simulink model "pet_logical_architecture"  (R2024a)
settings: Solver=FixedStepDiscrete  StartTime=0.0  StopTime=10.0  RelTol=1e-3
settings Model: Creator=diell  LastModifiedBy=diell

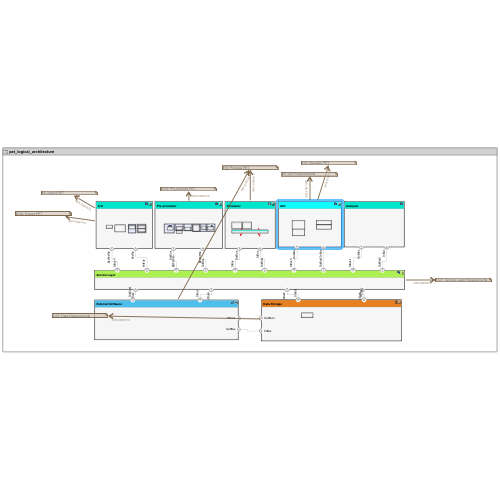
[thumbnail: Simulink's stored preview of the top-level diagram]
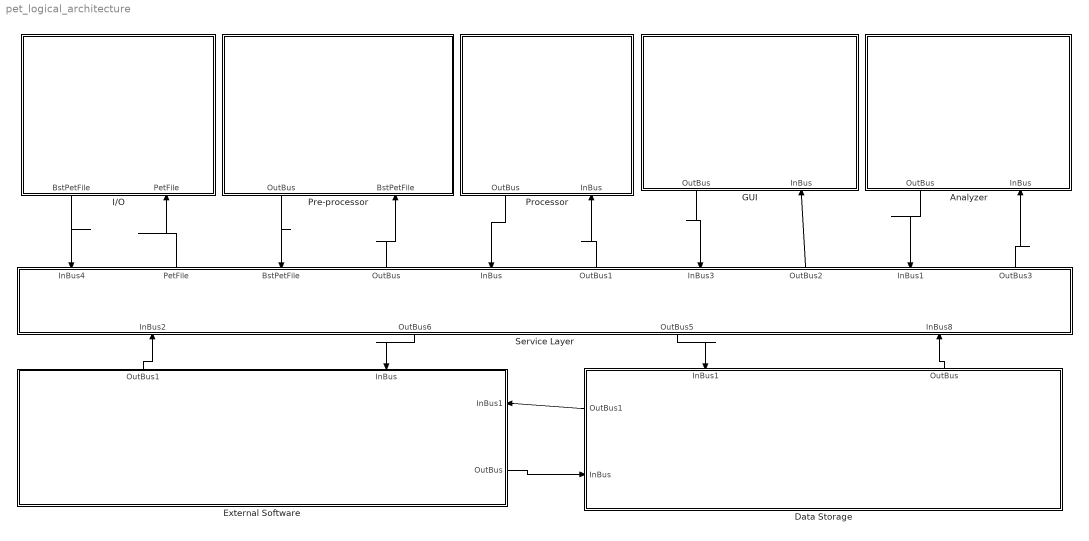
== system pet_logical_architecture ==
  Analyzer : Subsystem
      settings: PortSchema="{\"entries\":[{\"content\":{\"headerSize\":26,\"margin\":15,\"minimumSpacing\":25,\"sides\":[{\"content\":{},\"type\":\"ConnectorPlacement.EquallySpacedRectSide\",\"uuid\":\"231a4a51-e9d6-4ee1-a9d5-4e29b655c305\"},{\"content\":{\"side\":\"RIGHT\"},\"type\":\"ConnectorPlacement.EquallySpacedRectSide\",\"uuid\":\"e9ceff5f-0784-495f-ae83-524709d043d6\"},{\"content\":{\"side\":\"TOP\"},\"type\":\"ConnectorPlacement.EquallySpacedRectSide\",\"uuid\":\"01c193fb-23d5-46fa-9f50-f56eecaefc77\"},{\"content\":{\"connectorIds\":[\"Out1\",\"In1\"],\"side\":\"BOTTOM\"},\"type\":\"ConnectorPlacement.EquallySpacedRectSide\",\"uuid\":\"6027dc84-36e6-4171-8066-96bc152a4b70\"}]},\"type\":\"ConnectorPlacement.EquallySpacedConnector\",\"uuid\":\"bc597724-759a-481a-a480-4165a84a707f\"}],\"packageUris\":[\"http://schema.mathworks.com/mf0/Connector/R2020b\"],\"version\":\"1.0\"}"
  Data Storage : Subsystem
      settings: PortSchema="{\"entries\":[{\"content\":{\"headerSize\":26,\"margin\":15,\"minimumSpacing\":25,\"sides\":[{\"content\":{\"connectorIds\":[\"Out1\",\"In1\"]},\"type\":\"ConnectorPlacement.EquallySpacedRectSide\",\"uuid\":\"231a4a51-e9d6-4ee1-a9d5-4e29b655c305\"},{\"content\":{\"side\":\"RIGHT\"},\"type\":\"ConnectorPlacement.EquallySpacedRectSide\",\"uuid\":\"e9ceff5f-0784-495f-ae83-524709d043d6\"},{\"content\":{\"connectorIds\":[\"In2\",\"Out2\"],\"side\":\"TOP\"},\"type\":\"ConnectorPlacement.EquallySpacedRectSide\",\"uuid\":\"01c193fb-23d5-46fa-9f50-f56eecaefc77\"}]},\"type\":\"ConnectorPlacement.EquallySpacedConnector\",\"uuid\":\"bc597724-759a-481a-a480-4165a84a707f\"}],\"packageUris\":[\"http://schema.mathworks.com/mf0/Connector/R2020b\"],\"version\":\"1.0\"}"
  External Software : Subsystem
      settings: PortSchema="{\"entries\":[{\"content\":{\"headerSize\":26,\"margin\":15,\"minimumSpacing\":25,\"sides\":[{\"content\":{},\"type\":\"ConnectorPlacement.EquallySpacedRectSide\",\"uuid\":\"231a4a51-e9d6-4ee1-a9d5-4e29b655c305\"},{\"content\":{\"connectorIds\":[\"In1\",\"Out1\"],\"side\":\"RIGHT\"},\"type\":\"ConnectorPlacement.EquallySpacedRectSide\",\"uuid\":\"e9ceff5f-0784-495f-ae83-524709d043d6\"},{\"content\":{\"connectorIds\":[\"Out2\",\"In2\"],\"side\":\"TOP\"},\"type\":\"ConnectorPlacement.EquallySpacedRectSide\",\"uuid\":\"01c193fb-23d5-46fa-9f50-f56eecaefc77\"}]},\"type\":\"ConnectorPlacement.EquallySpacedConnector\",\"uuid\":\"bc597724-759a-481a-a480-4165a84a707f\"}],\"packageUris\":[\"http://schema.mathworks.com/mf0/Connector/R2020b\"],\"version\":\"1.0\"}"
  GUI : Subsystem
      settings: PortSchema="{\"entries\":[{\"content\":{\"headerSize\":26,\"margin\":15,\"minimumSpacing\":25,\"sides\":[{\"content\":{},\"type\":\"ConnectorPlacement.EquallySpacedRectSide\",\"uuid\":\"231a4a51-e9d6-4ee1-a9d5-4e29b655c305\"},{\"content\":{\"side\":\"RIGHT\"},\"type\":\"ConnectorPlacement.EquallySpacedRectSide\",\"uuid\":\"e9ceff5f-0784-495f-ae83-524709d043d6\"},{\"content\":{\"side\":\"TOP\"},\"type\":\"ConnectorPlacement.EquallySpacedRectSide\",\"uuid\":\"01c193fb-23d5-46fa-9f50-f56eecaefc77\"},{\"content\":{\"connectorIds\":[\"Out1\",\"In1\"],\"side\":\"BOTTOM\"},\"type\":\"ConnectorPlacement.EquallySpacedRectSide\",\"uuid\":\"8789287b-37dd-46ec-841a-db569d1bc1a9\"}]},\"type\":\"ConnectorPlacement.EquallySpacedConnector\",\"uuid\":\"bc597724-759a-481a-a480-4165a84a707f\"}],\"packageUris\":[\"http://schema.mathworks.com/mf0/Connector/R2020b\"],\"version\":\"1.0\"}"
  "I/O " : Subsystem
      settings: PortSchema="{\"entries\":[{\"content\":{\"headerSize\":26,\"margin\":15,\"minimumSpacing\":25,\"sides\":[{\"content\":{},\"type\":\"ConnectorPlacement.EquallySpacedRectSide\",\"uuid\":\"231a4a51-e9d6-4ee1-a9d5-4e29b655c305\"},{\"content\":{\"side\":\"RIGHT\"},\"type\":\"ConnectorPlacement.EquallySpacedRectSide\",\"uuid\":\"e9ceff5f-0784-495f-ae83-524709d043d6\"},{\"content\":{\"side\":\"TOP\"},\"type\":\"ConnectorPlacement.EquallySpacedRectSide\",\"uuid\":\"01c193fb-23d5-46fa-9f50-f56eecaefc77\"},{\"content\":{\"connectorIds\":[\"Out1\",\"In1\"],\"side\":\"BOTTOM\"},\"type\":\"ConnectorPlacement.EquallySpacedRectSide\",\"uuid\":\"53c8788b-6d16-4a86-bf5b-c8def0072bdd\"}]},\"type\":\"ConnectorPlacement.EquallySpacedConnector\",\"uuid\":\"bc597724-759a-481a-a480-4165a84a707f\"}],\"packageUris\":[\"http://schema.mathworks.com/mf0/Connector/R2020b\"],\"version\":\"1.0\"}"
  Pre-processor : Subsystem
      settings: PortSchema="{\"entries\":[{\"content\":{\"headerSize\":26,\"margin\":15,\"minimumSpacing\":25,\"sides\":[{\"content\":{},\"type\":\"ConnectorPlacement.EquallySpacedRectSide\",\"uuid\":\"231a4a51-e9d6-4ee1-a9d5-4e29b655c305\"},{\"content\":{\"side\":\"RIGHT\"},\"type\":\"ConnectorPlacement.EquallySpacedRectSide\",\"uuid\":\"e9ceff5f-0784-495f-ae83-524709d043d6\"},{\"content\":{\"side\":\"TOP\"},\"type\":\"ConnectorPlacement.EquallySpacedRectSide\",\"uuid\":\"01c193fb-23d5-46fa-9f50-f56eecaefc77\"},{\"content\":{\"connectorIds\":[\"Out1\",\"In1\"],\"side\":\"BOTTOM\"},\"type\":\"ConnectorPlacement.EquallySpacedRectSide\",\"uuid\":\"b0b0d034-7ae8-4ce9-aa3d-1431a9441512\"}]},\"type\":\"ConnectorPlacement.EquallySpacedConnector\",\"uuid\":\"bc597724-759a-481a-a480-4165a84a707f\"}],\"packageUris\":[\"http://schema.mathworks.com/mf0/Connector/R2020b\"],\"version\":\"1.0\"}"
  Processor : Subsystem
      settings: PortSchema="{\"entries\":[{\"content\":{\"headerSize\":26,\"margin\":15,\"minimumSpacing\":25,\"sides\":[{\"content\":{},\"type\":\"ConnectorPlacement.EquallySpacedRectSide\",\"uuid\":\"231a4a51-e9d6-4ee1-a9d5-4e29b655c305\"},{\"content\":{\"side\":\"RIGHT\"},\"type\":\"ConnectorPlacement.EquallySpacedRectSide\",\"uuid\":\"e9ceff5f-0784-495f-ae83-524709d043d6\"},{\"content\":{\"side\":\"TOP\"},\"type\":\"ConnectorPlacement.EquallySpacedRectSide\",\"uuid\":\"01c193fb-23d5-46fa-9f50-f56eecaefc77\"},{\"content\":{\"connectorIds\":[\"Out1\",\"In1\"],\"side\":\"BOTTOM\"},\"type\":\"ConnectorPlacement.EquallySpacedRectSide\",\"uuid\":\"096d348b-1de6-4ed0-877f-8a116cb4ec66\"}]},\"type\":\"ConnectorPlacement.EquallySpacedConnector\",\"uuid\":\"bc597724-759a-481a-a480-4165a84a707f\"}],\"packageUris\":[\"http://schema.mathworks.com/mf0/Connector/R2020b\"],\"version\":\"1.0\"}"
  Service Layer : Subsystem
      settings: PortSchema="{\"entries\":[{\"content\":{\"headerSize\":26,\"margin\":15,\"minimumSpacing\":25,\"sides\":[{\"content\":{},\"type\":\"ConnectorPlacement.EquallySpacedRectSide\",\"uuid\":\"231a4a51-e9d6-4ee1-a9d5-4e29b655c305\"},{\"content\":{\"side\":\"RIGHT\"},\"type\":\"ConnectorPlacement.EquallySpacedRectSide\",\"uuid\":\"e9ceff5f-0784-495f-ae83-524709d043d6\"},{\"content\":{\"connectorIds\":[\"In1\",\"Out1\",\"In5\",\"Out3\",\"In2\",\"Out2\",\"In3\",\"Out4\",\"In4\",\"Out5\"],\"side\":\"TOP\"},\"type\":\"ConnectorPlacement.EquallySpacedRectSide\",\"uuid\":\"01c193fb-23d5-46fa-9f50-f56eecaefc77\"},{\"content\":{\"connectorIds\":[\"In6\",\"Out6\",\"Out7\",\"In7\"],\"side\":\"BOTTOM\"},\"type\":\"ConnectorPlacement.EquallySpacedRectSide\",\"uuid\":\"8a7a1846-1a54-4dcd-b18c-069e384b1e61\"}]},\"type\":\"ConnectorPlacement.EquallySpacedConnector\",\"uuid\":\"bc597724-759a-481a-a480-4165a84a707f\"}],\"packageUris\":[\"http://schema.mathworks.com/mf0/Connector/R2020b\"],\"version\":\"1.0\"}"
  wires:
  Data Storage/2(OutBus) -> Service Layer/7(InBus8)
  Service Layer/7(OutBus5) -> Data Storage/2(InBus1)
  Service Layer/6(OutBus6) -> External Software/2(InBus)
  External Software/2(OutBus1) -> Service Layer/6(InBus2)
  External Software/1(OutBus) -> Data Storage/1(InBus)
  Data Storage/1(OutBus1) -> External Software/1(InBus1)
  Service Layer/1(PetFile) -> "I/O "/1(PetFile)
  Pre-processor/1(OutBus) -> Service Layer/5(BstPetFile)
  Service Layer/3(OutBus) -> Pre-processor/1(BstPetFile)
  Processor/1(OutBus) -> Service Layer/2(InBus)
  Service Layer/2(OutBus1) -> Processor/1(InBus)
  GUI/1(OutBus) -> Service Layer/3(InBus3)
  Service Layer/4(OutBus2) -> GUI/1(InBus)
  Analyzer/1(OutBus) -> Service Layer/4(InBus1)
  Service Layer/5(OutBus3) -> Analyzer/1(InBus)
  "I/O "/1(BstPetFile) -> Service Layer/1(InBus4)

== system pet_logical_architecture/Analyzer ==
  Bus Element In1 : Inport  PortName=InBus
  Bus Element Out1 : Outport  PortName=OutBus

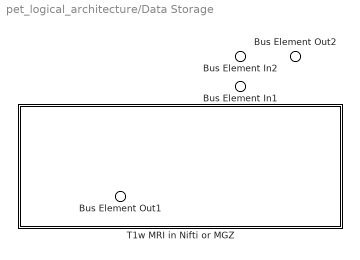
== system pet_logical_architecture/Data Storage ==
  Bus Element In1 : Inport  PortName=InBus
  Bus Element In2 : Inport  Port=2  PortName=InBus1
  T1w MRI in Nifti or MGZ : Subsystem
      settings: PortSchema="{\"entries\":[{\"content\":{\"headerSize\":26,\"margin\":15,\"minimumSpacing\":25,\"sides\":[{\"content\":{},\"type\":\"ConnectorPlacement.EquallySpacedRectSide\",\"uuid\":\"41d3ebd7-d990-4c64-a8fe-a1444a13acba\"},{\"content\":{\"side\":\"RIGHT\"},\"type\":\"ConnectorPlacement.EquallySpacedRectSide\",\"uuid\":\"34a032e5-8bdc-4c16-a398-56e9e8002181\"},{\"content\":{\"side\":\"TOP\"},\"type\":\"ConnectorPlacement.EquallySpacedRectSide\",\"uuid\":\"d28171cf-e891-45d3-8ea9-b10c38c32c2e\"}]},\"type\":\"ConnectorPlacement.EquallySpacedConnector\",\"uuid\":\"0daa939b-8979-496f-bab9-c42cbb494216\"}],\"packageUris\":[\"http://schema.mathworks.com/mf0/Connector/R2020b\"],\"version\":\"1.0\"}"
  Bus Element Out2 : Outport  PortName=OutBus1
  Bus Element Out1 : Outport  Port=2  PortName=OutBus

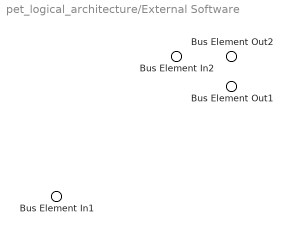
== system pet_logical_architecture/External Software ==
  Bus Element In2 : Inport  PortName=InBus1
  Bus Element In1 : Inport  Port=2  PortName=InBus
  Bus Element Out1 : Outport  PortName=OutBus
  Bus Element Out2 : Outport  Port=2  PortName=OutBus1

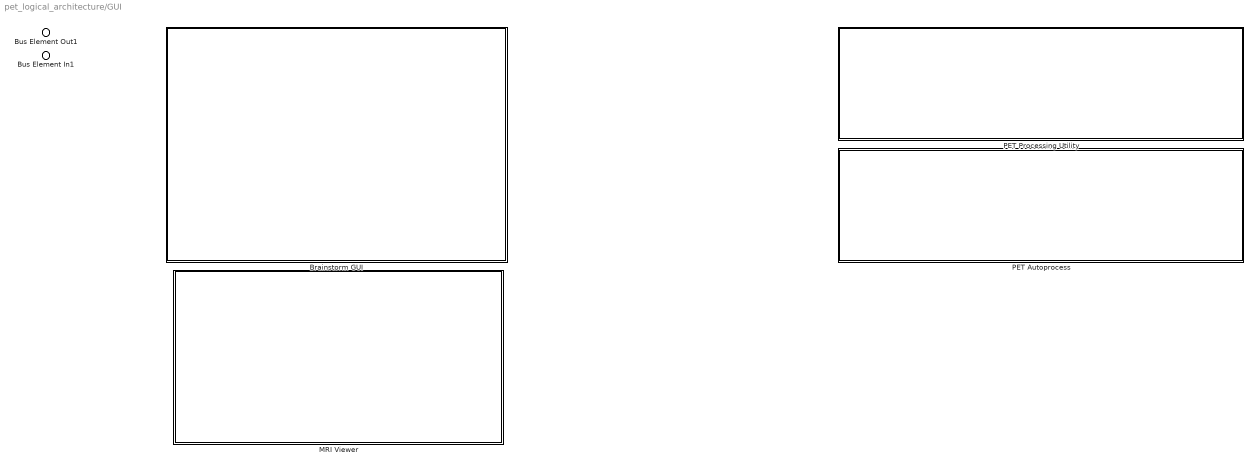
== system pet_logical_architecture/GUI ==
  Bus Element In1 : Inport  PortName=InBus
  "Brainstorm GUI " : Subsystem
      settings: PortSchema="{\"entries\":[{\"content\":{\"headerSize\":26,\"margin\":15,\"minimumSpacing\":25,\"sides\":[{\"content\":{},\"type\":\"ConnectorPlacement.EquallySpacedRectSide\",\"uuid\":\"41d3ebd7-d990-4c64-a8fe-a1444a13acba\"},{\"content\":{\"side\":\"RIGHT\"},\"type\":\"ConnectorPlacement.EquallySpacedRectSide\",\"uuid\":\"34a032e5-8bdc-4c16-a398-56e9e8002181\"},{\"content\":{\"side\":\"TOP\"},\"type\":\"ConnectorPlacement.EquallySpacedRectSide\",\"uuid\":\"d28171cf-e891-45d3-8ea9-b10c38c32c2e\"}]},\"type\":\"ConnectorPlacement.EquallySpacedConnector\",\"uuid\":\"0daa939b-8979-496f-bab9-c42cbb494216\"}],\"packageUris\":[\"http://schema.mathworks.com/mf0/Connector/R2020b\"],\"version\":\"1.0\"}"
  MRI Viewer : Subsystem
      settings: PortSchema="{\"entries\":[{\"content\":{\"headerSize\":26,\"margin\":15,\"minimumSpacing\":25,\"sides\":[{\"content\":{},\"type\":\"ConnectorPlacement.EquallySpacedRectSide\",\"uuid\":\"41d3ebd7-d990-4c64-a8fe-a1444a13acba\"},{\"content\":{\"side\":\"RIGHT\"},\"type\":\"ConnectorPlacement.EquallySpacedRectSide\",\"uuid\":\"34a032e5-8bdc-4c16-a398-56e9e8002181\"},{\"content\":{\"side\":\"TOP\"},\"type\":\"ConnectorPlacement.EquallySpacedRectSide\",\"uuid\":\"d28171cf-e891-45d3-8ea9-b10c38c32c2e\"}]},\"type\":\"ConnectorPlacement.EquallySpacedConnector\",\"uuid\":\"0daa939b-8979-496f-bab9-c42cbb494216\"}],\"packageUris\":[\"http://schema.mathworks.com/mf0/Connector/R2020b\"],\"version\":\"1.0\"}"
  PET Autoprocess : Subsystem
      settings: PortSchema="{\"entries\":[{\"content\":{\"headerSize\":26,\"margin\":15,\"minimumSpacing\":25,\"sides\":[{\"content\":{},\"type\":\"ConnectorPlacement.EquallySpacedRectSide\",\"uuid\":\"41d3ebd7-d990-4c64-a8fe-a1444a13acba\"},{\"content\":{\"side\":\"RIGHT\"},\"type\":\"ConnectorPlacement.EquallySpacedRectSide\",\"uuid\":\"34a032e5-8bdc-4c16-a398-56e9e8002181\"},{\"content\":{\"side\":\"TOP\"},\"type\":\"ConnectorPlacement.EquallySpacedRectSide\",\"uuid\":\"d28171cf-e891-45d3-8ea9-b10c38c32c2e\"}]},\"type\":\"ConnectorPlacement.EquallySpacedConnector\",\"uuid\":\"0daa939b-8979-496f-bab9-c42cbb494216\"}],\"packageUris\":[\"http://schema.mathworks.com/mf0/Connector/R2020b\"],\"version\":\"1.0\"}"
  PET Processing Utility : Subsystem
      settings: PortSchema="{\"entries\":[{\"content\":{\"headerSize\":26,\"margin\":15,\"minimumSpacing\":25,\"sides\":[{\"content\":{},\"type\":\"ConnectorPlacement.EquallySpacedRectSide\",\"uuid\":\"41d3ebd7-d990-4c64-a8fe-a1444a13acba\"},{\"content\":{\"side\":\"RIGHT\"},\"type\":\"ConnectorPlacement.EquallySpacedRectSide\",\"uuid\":\"34a032e5-8bdc-4c16-a398-56e9e8002181\"},{\"content\":{\"side\":\"TOP\"},\"type\":\"ConnectorPlacement.EquallySpacedRectSide\",\"uuid\":\"d28171cf-e891-45d3-8ea9-b10c38c32c2e\"}]},\"type\":\"ConnectorPlacement.EquallySpacedConnector\",\"uuid\":\"0daa939b-8979-496f-bab9-c42cbb494216\"}],\"packageUris\":[\"http://schema.mathworks.com/mf0/Connector/R2020b\"],\"version\":\"1.0\"}"
  Bus Element Out1 : Outport  PortName=OutBus

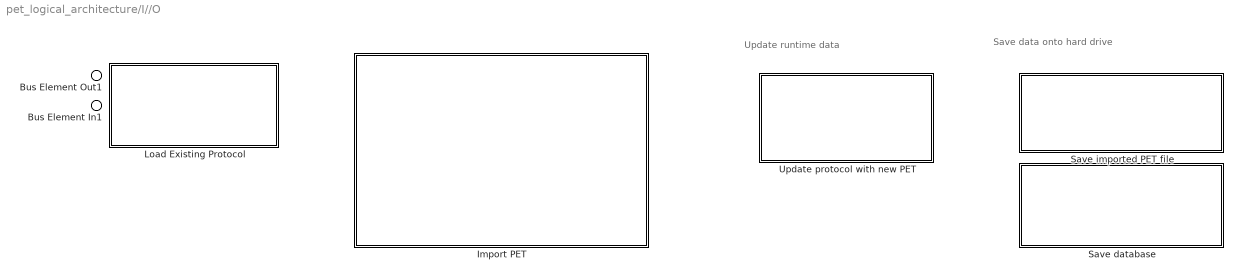
== system pet_logical_architecture/I//O  ==
  note: Save data onto hard drive
  note: Update runtime data
  Bus Element In1 : Inport  PortName=PetFile
  Import PET : Subsystem
      settings: PortSchema="{\"entries\":[{\"content\":{\"headerSize\":26,\"margin\":15,\"minimumSpacing\":25,\"sides\":[{\"content\":{},\"type\":\"ConnectorPlacement.EquallySpacedRectSide\",\"uuid\":\"9a42c3ee-f5d5-46c5-b9f0-29e49ed7c7b7\"},{\"content\":{\"side\":\"RIGHT\"},\"type\":\"ConnectorPlacement.EquallySpacedRectSide\",\"uuid\":\"669ba6ca-2a72-430e-84d2-b9b4202c74ab\"},{\"content\":{\"side\":\"TOP\"},\"type\":\"ConnectorPlacement.EquallySpacedRectSide\",\"uuid\":\"659c07dc-ee6b-4566-a70e-b6beb842b74e\"}]},\"type\":\"ConnectorPlacement.EquallySpacedConnector\",\"uuid\":\"e9499bf4-698a-44d7-8b3a-a6a8c827afce\"}],\"packageUris\":[\"http://schema.mathworks.com/mf0/Connector/R2020b\"],\"version\":\"1.0\"}"
  Load Existing Protocol : Subsystem
      settings: PortSchema="{\"entries\":[{\"content\":{\"headerSize\":26,\"margin\":15,\"minimumSpacing\":25,\"sides\":[{\"content\":{},\"type\":\"ConnectorPlacement.EquallySpacedRectSide\",\"uuid\":\"9a42c3ee-f5d5-46c5-b9f0-29e49ed7c7b7\"},{\"content\":{\"side\":\"RIGHT\"},\"type\":\"ConnectorPlacement.EquallySpacedRectSide\",\"uuid\":\"669ba6ca-2a72-430e-84d2-b9b4202c74ab\"},{\"content\":{\"side\":\"TOP\"},\"type\":\"ConnectorPlacement.EquallySpacedRectSide\",\"uuid\":\"659c07dc-ee6b-4566-a70e-b6beb842b74e\"}]},\"type\":\"ConnectorPlacement.EquallySpacedConnector\",\"uuid\":\"e9499bf4-698a-44d7-8b3a-a6a8c827afce\"}],\"packageUris\":[\"http://schema.mathworks.com/mf0/Connector/R2020b\"],\"version\":\"1.0\"}"
  Save database : Subsystem
      settings: PortSchema="{\"entries\":[{\"content\":{\"headerSize\":26,\"margin\":15,\"minimumSpacing\":25,\"sides\":[{\"content\":{},\"type\":\"ConnectorPlacement.EquallySpacedRectSide\",\"uuid\":\"9a42c3ee-f5d5-46c5-b9f0-29e49ed7c7b7\"},{\"content\":{\"side\":\"RIGHT\"},\"type\":\"ConnectorPlacement.EquallySpacedRectSide\",\"uuid\":\"669ba6ca-2a72-430e-84d2-b9b4202c74ab\"},{\"content\":{\"side\":\"TOP\"},\"type\":\"ConnectorPlacement.EquallySpacedRectSide\",\"uuid\":\"659c07dc-ee6b-4566-a70e-b6beb842b74e\"}]},\"type\":\"ConnectorPlacement.EquallySpacedConnector\",\"uuid\":\"e9499bf4-698a-44d7-8b3a-a6a8c827afce\"}],\"packageUris\":[\"http://schema.mathworks.com/mf0/Connector/R2020b\"],\"version\":\"1.0\"}"
  Save imported PET file : Subsystem
      settings: PortSchema="{\"entries\":[{\"content\":{\"headerSize\":26,\"margin\":15,\"minimumSpacing\":25,\"sides\":[{\"content\":{},\"type\":\"ConnectorPlacement.EquallySpacedRectSide\",\"uuid\":\"9a42c3ee-f5d5-46c5-b9f0-29e49ed7c7b7\"},{\"content\":{\"side\":\"RIGHT\"},\"type\":\"ConnectorPlacement.EquallySpacedRectSide\",\"uuid\":\"669ba6ca-2a72-430e-84d2-b9b4202c74ab\"},{\"content\":{\"side\":\"TOP\"},\"type\":\"ConnectorPlacement.EquallySpacedRectSide\",\"uuid\":\"659c07dc-ee6b-4566-a70e-b6beb842b74e\"}]},\"type\":\"ConnectorPlacement.EquallySpacedConnector\",\"uuid\":\"e9499bf4-698a-44d7-8b3a-a6a8c827afce\"}],\"packageUris\":[\"http://schema.mathworks.com/mf0/Connector/R2020b\"],\"version\":\"1.0\"}"
  Update protocol with new PET : Subsystem
      settings: PortSchema="{\"entries\":[{\"content\":{\"headerSize\":26,\"margin\":15,\"minimumSpacing\":25,\"sides\":[{\"content\":{},\"type\":\"ConnectorPlacement.EquallySpacedRectSide\",\"uuid\":\"9a42c3ee-f5d5-46c5-b9f0-29e49ed7c7b7\"},{\"content\":{\"side\":\"RIGHT\"},\"type\":\"ConnectorPlacement.EquallySpacedRectSide\",\"uuid\":\"669ba6ca-2a72-430e-84d2-b9b4202c74ab\"},{\"content\":{\"side\":\"TOP\"},\"type\":\"ConnectorPlacement.EquallySpacedRectSide\",\"uuid\":\"659c07dc-ee6b-4566-a70e-b6beb842b74e\"},{\"content\":{\"side\":\"BOTTOM\"},\"type\":\"ConnectorPlacement.EquallySpacedRectSide\",\"uuid\":\"cf282e21-1e43-4117-abb4-23de90c90cc3\"}]},\"type\":\"ConnectorPlacement.EquallySpacedConnector\",\"uuid\":\"e9499bf4-698a-44d7-8b3a-a6a8c827afce\"}],\"packageUris\":[\"http://schema.mathworks.com/mf0/Connector/R2020b\"],\"version\":\"1.0\"}"
  Bus Element Out1 : Outport  PortName=BstPetFile

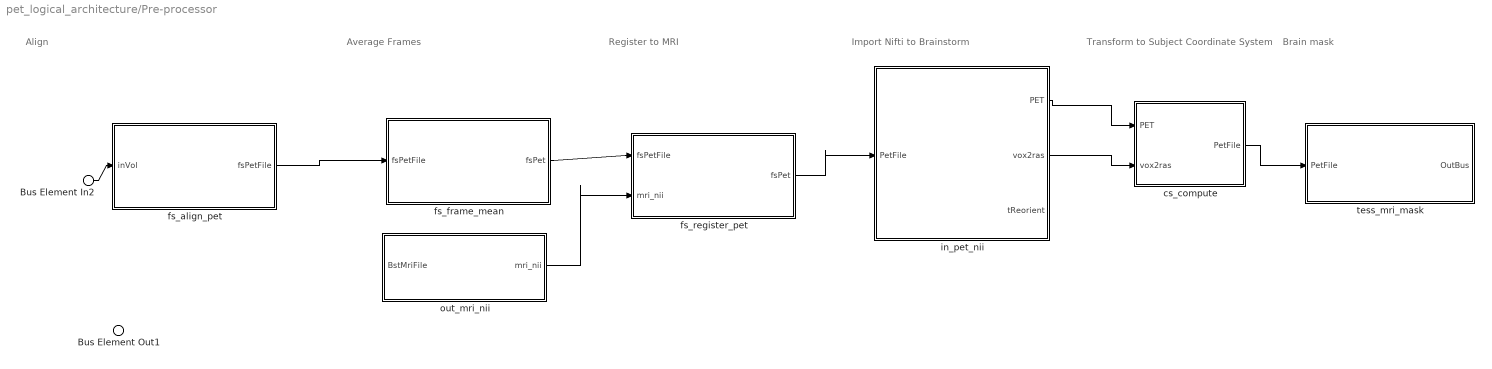
== system pet_logical_architecture/Pre-processor ==
  note: Align
  note: Average Frames
  note: Transform to
      | Subject Coordinate System
  note: Register to MRI
  note: Brain mask
  note: Import Nifti to Brainstorm
  Bus Element In2 : Inport  PortName=BstPetFile
  cs_compute : Subsystem
      settings: PortSchema="{\"entries\":[{\"content\":{\"headerSize\":26,\"margin\":15,\"minimumSpacing\":25,\"sides\":[{\"content\":{\"connectorIds\":[\"In1\",\"In2\"]},\"type\":\"ConnectorPlacement.EquallySpacedRectSide\",\"uuid\":\"d9face5b-155e-4e83-95c0-d581b737b6e3\"},{\"content\":{\"connectorIds\":[\"Out1\"],\"side\":\"RIGHT\"},\"type\":\"ConnectorPlacement.EquallySpacedRectSide\",\"uuid\":\"f965be1f-1639-4140-b9ea-f5e9efbe4150\"},{\"content\":{\"side\":\"TOP\"},\"type\":\"ConnectorPlacement.EquallySpacedRectSide\",\"uuid\":\"7c9c4b2b-011c-4482-afab-b6e67025a5e2\"}]},\"type\":\"ConnectorPlacement.EquallySpacedConnector\",\"uuid\":\"ec963004-117d-4f22-bb00-71f35201e6e2\"}],\"packageUris\":[\"http://schema.mathworks.com/mf0/Connector/R2020b\"],\"version\":\"1.0\"}"
  fs_align_pet : Subsystem
      settings: PortSchema="{\"entries\":[{\"content\":{\"headerSize\":26,\"margin\":15,\"minimumSpacing\":25,\"sides\":[{\"content\":{\"connectorIds\":[\"In1\"]},\"type\":\"ConnectorPlacement.EquallySpacedRectSide\",\"uuid\":\"d9face5b-155e-4e83-95c0-d581b737b6e3\"},{\"content\":{\"connectorIds\":[\"Out1\"],\"side\":\"RIGHT\"},\"type\":\"ConnectorPlacement.EquallySpacedRectSide\",\"uuid\":\"f965be1f-1639-4140-b9ea-f5e9efbe4150\"},{\"content\":{\"side\":\"TOP\"},\"type\":\"ConnectorPlacement.EquallySpacedRectSide\",\"uuid\":\"7c9c4b2b-011c-4482-afab-b6e67025a5e2\"}]},\"type\":\"ConnectorPlacement.EquallySpacedConnector\",\"uuid\":\"ec963004-117d-4f22-bb00-71f35201e6e2\"}],\"packageUris\":[\"http://schema.mathworks.com/mf0/Connector/R2020b\"],\"version\":\"1.0\"}"
  fs_frame_mean : Subsystem
      settings: PortSchema="{\"entries\":[{\"content\":{\"headerSize\":26,\"margin\":15,\"minimumSpacing\":25,\"sides\":[{\"content\":{\"connectorIds\":[\"In1\"]},\"type\":\"ConnectorPlacement.EquallySpacedRectSide\",\"uuid\":\"d9face5b-155e-4e83-95c0-d581b737b6e3\"},{\"content\":{\"connectorIds\":[\"Out1\"],\"side\":\"RIGHT\"},\"type\":\"ConnectorPlacement.EquallySpacedRectSide\",\"uuid\":\"f965be1f-1639-4140-b9ea-f5e9efbe4150\"},{\"content\":{\"side\":\"TOP\"},\"type\":\"ConnectorPlacement.EquallySpacedRectSide\",\"uuid\":\"7c9c4b2b-011c-4482-afab-b6e67025a5e2\"}]},\"type\":\"ConnectorPlacement.EquallySpacedConnector\",\"uuid\":\"ec963004-117d-4f22-bb00-71f35201e6e2\"}],\"packageUris\":[\"http://schema.mathworks.com/mf0/Connector/R2020b\"],\"version\":\"1.0\"}"
  fs_register_pet : Subsystem
      settings: PortSchema="{\"entries\":[{\"content\":{\"headerSize\":26,\"margin\":15,\"minimumSpacing\":25,\"sides\":[{\"content\":{\"connectorIds\":[\"In1\",\"In2\"]},\"type\":\"ConnectorPlacement.EquallySpacedRectSide\",\"uuid\":\"d9face5b-155e-4e83-95c0-d581b737b6e3\"},{\"content\":{\"connectorIds\":[\"Out1\"],\"side\":\"RIGHT\"},\"type\":\"ConnectorPlacement.EquallySpacedRectSide\",\"uuid\":\"f965be1f-1639-4140-b9ea-f5e9efbe4150\"},{\"content\":{\"side\":\"TOP\"},\"type\":\"ConnectorPlacement.EquallySpacedRectSide\",\"uuid\":\"7c9c4b2b-011c-4482-afab-b6e67025a5e2\"}]},\"type\":\"ConnectorPlacement.EquallySpacedConnector\",\"uuid\":\"ec963004-117d-4f22-bb00-71f35201e6e2\"}],\"packageUris\":[\"http://schema.mathworks.com/mf0/Connector/R2020b\"],\"version\":\"1.0\"}"
  in_pet_nii : Subsystem
      settings: PortSchema="{\"entries\":[{\"content\":{\"headerSize\":26,\"margin\":15,\"minimumSpacing\":25,\"sides\":[{\"content\":{\"connectorIds\":[\"In1\"]},\"type\":\"ConnectorPlacement.EquallySpacedRectSide\",\"uuid\":\"d9face5b-155e-4e83-95c0-d581b737b6e3\"},{\"content\":{\"connectorIds\":[\"Out1\",\"Out2\",\"Out3\"],\"side\":\"RIGHT\"},\"type\":\"ConnectorPlacement.EquallySpacedRectSide\",\"uuid\":\"f965be1f-1639-4140-b9ea-f5e9efbe4150\"},{\"content\":{\"side\":\"TOP\"},\"type\":\"ConnectorPlacement.EquallySpacedRectSide\",\"uuid\":\"7c9c4b2b-011c-4482-afab-b6e67025a5e2\"}]},\"type\":\"ConnectorPlacement.EquallySpacedConnector\",\"uuid\":\"ec963004-117d-4f22-bb00-71f35201e6e2\"}],\"packageUris\":[\"http://schema.mathworks.com/mf0/Connector/R2020b\"],\"version\":\"1.0\"}"
  out_mri_nii : Subsystem
      settings: PortSchema="{\"entries\":[{\"content\":{\"headerSize\":26,\"margin\":15,\"minimumSpacing\":25,\"sides\":[{\"content\":{\"connectorIds\":[\"In1\"]},\"type\":\"ConnectorPlacement.EquallySpacedRectSide\",\"uuid\":\"d9face5b-155e-4e83-95c0-d581b737b6e3\"},{\"content\":{\"connectorIds\":[\"Out1\"],\"side\":\"RIGHT\"},\"type\":\"ConnectorPlacement.EquallySpacedRectSide\",\"uuid\":\"f965be1f-1639-4140-b9ea-f5e9efbe4150\"},{\"content\":{\"side\":\"TOP\"},\"type\":\"ConnectorPlacement.EquallySpacedRectSide\",\"uuid\":\"7c9c4b2b-011c-4482-afab-b6e67025a5e2\"}]},\"type\":\"ConnectorPlacement.EquallySpacedConnector\",\"uuid\":\"ec963004-117d-4f22-bb00-71f35201e6e2\"}],\"packageUris\":[\"http://schema.mathworks.com/mf0/Connector/R2020b\"],\"version\":\"1.0\"}"
  tess_mri_mask : Subsystem
      settings: PortSchema="{\"entries\":[{\"content\":{\"headerSize\":26,\"margin\":15,\"minimumSpacing\":25,\"sides\":[{\"content\":{\"connectorIds\":[\"In1\"]},\"type\":\"ConnectorPlacement.EquallySpacedRectSide\",\"uuid\":\"d9face5b-155e-4e83-95c0-d581b737b6e3\"},{\"content\":{\"connectorIds\":[\"Out1\"],\"side\":\"RIGHT\"},\"type\":\"ConnectorPlacement.EquallySpacedRectSide\",\"uuid\":\"f965be1f-1639-4140-b9ea-f5e9efbe4150\"},{\"content\":{\"side\":\"TOP\"},\"type\":\"ConnectorPlacement.EquallySpacedRectSide\",\"uuid\":\"7c9c4b2b-011c-4482-afab-b6e67025a5e2\"}]},\"type\":\"ConnectorPlacement.EquallySpacedConnector\",\"uuid\":\"ec963004-117d-4f22-bb00-71f35201e6e2\"}],\"packageUris\":[\"http://schema.mathworks.com/mf0/Connector/R2020b\"],\"version\":\"1.0\"}"
  Bus Element Out1 : Outport  PortName=OutBus
  wires:
  in_pet_nii/1(PET) -> cs_compute/1(PET)
  fs_register_pet/1(fsPet) -> in_pet_nii/1(PetFile)
  Bus Element In2/1 -> fs_align_pet/1(inVol)
  in_pet_nii/2(vox2ras) -> cs_compute/2(vox2ras)
  cs_compute/1(PetFile) -> tess_mri_mask/1(PetFile)
  fs_frame_mean/1(fsPet) -> fs_register_pet/1(fsPetFile)
  out_mri_nii/1(mri_nii) -> fs_register_pet/2(mri_nii)
  fs_align_pet/1(fsPetFile) -> fs_frame_mean/1(fsPetFile)

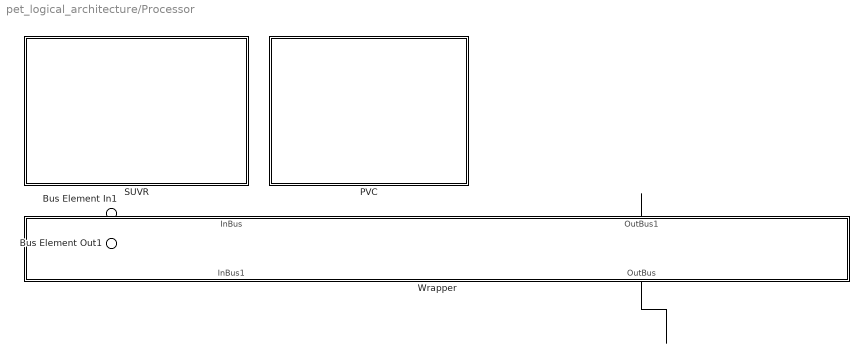
== system pet_logical_architecture/Processor ==
  Bus Element In1 : Inport  PortName=InBus
  "PVC " : Subsystem
      settings: PortSchema="{\"entries\":[{\"content\":{\"headerSize\":26,\"margin\":15,\"minimumSpacing\":25,\"sides\":[{\"content\":{},\"type\":\"ConnectorPlacement.EquallySpacedRectSide\",\"uuid\":\"231a4a51-e9d6-4ee1-a9d5-4e29b655c305\"},{\"content\":{\"side\":\"RIGHT\"},\"type\":\"ConnectorPlacement.EquallySpacedRectSide\",\"uuid\":\"e9ceff5f-0784-495f-ae83-524709d043d6\"},{\"content\":{\"side\":\"TOP\"},\"type\":\"ConnectorPlacement.EquallySpacedRectSide\",\"uuid\":\"01c193fb-23d5-46fa-9f50-f56eecaefc77\"}]},\"type\":\"ConnectorPlacement.EquallySpacedConnector\",\"uuid\":\"bc597724-759a-481a-a480-4165a84a707f\"}],\"packageUris\":[\"http://schema.mathworks.com/mf0/Connector/R2020b\"],\"version\":\"1.0\"}"
  SUVR : Subsystem
      settings: PortSchema="{\"entries\":[{\"content\":{\"headerSize\":26,\"margin\":15,\"minimumSpacing\":25,\"sides\":[{\"content\":{},\"type\":\"ConnectorPlacement.EquallySpacedRectSide\",\"uuid\":\"231a4a51-e9d6-4ee1-a9d5-4e29b655c305\"},{\"content\":{\"side\":\"RIGHT\"},\"type\":\"ConnectorPlacement.EquallySpacedRectSide\",\"uuid\":\"e9ceff5f-0784-495f-ae83-524709d043d6\"},{\"content\":{\"side\":\"TOP\"},\"type\":\"ConnectorPlacement.EquallySpacedRectSide\",\"uuid\":\"01c193fb-23d5-46fa-9f50-f56eecaefc77\"}]},\"type\":\"ConnectorPlacement.EquallySpacedConnector\",\"uuid\":\"bc597724-759a-481a-a480-4165a84a707f\"}],\"packageUris\":[\"http://schema.mathworks.com/mf0/Connector/R2020b\"],\"version\":\"1.0\"}"
  Wrapper : Subsystem
      settings: PortSchema="{\"entries\":[{\"content\":{\"headerSize\":26,\"margin\":15,\"minimumSpacing\":25,\"sides\":[{\"content\":{},\"type\":\"ConnectorPlacement.EquallySpacedRectSide\",\"uuid\":\"231a4a51-e9d6-4ee1-a9d5-4e29b655c305\"},{\"content\":{\"side\":\"RIGHT\"},\"type\":\"ConnectorPlacement.EquallySpacedRectSide\",\"uuid\":\"e9ceff5f-0784-495f-ae83-524709d043d6\"},{\"content\":{\"connectorIds\":[\"In1\",\"Out1\"],\"side\":\"TOP\"},\"type\":\"ConnectorPlacement.EquallySpacedRectSide\",\"uuid\":\"01c193fb-23d5-46fa-9f50-f56eecaefc77\"},{\"content\":{\"connectorIds\":[\"In2\",\"Out2\"],\"side\":\"BOTTOM\"},\"type\":\"ConnectorPlacement.EquallySpacedRectSide\",\"uuid\":\"1e15f760-b7da-470b-a846-203fd9acf6b7\"}]},\"type\":\"ConnectorPlacement.EquallySpacedConnector\",\"uuid\":\"bc597724-759a-481a-a480-4165a84a707f\"}],\"packageUris\":[\"http://schema.mathworks.com/mf0/Connector/R2020b\"],\"version\":\"1.0\"}"
  Bus Element Out1 : Outport  PortName=OutBus
  wires:
  ? -> Wrapper/2(InBus1)
  Wrapper/1(OutBus1) -> ?
  Wrapper/2(OutBus) -> ?
  ? -> Wrapper/1(InBus)

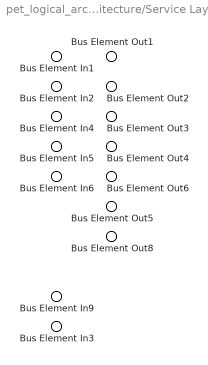
== system pet_logical_architecture/Service Layer ==
  Bus Element In6 : Inport  PortName=InBus4
  Bus Element In4 : Inport  Port=2  PortName=InBus
  Bus Element In5 : Inport  Port=3  PortName=InBus3
  Bus Element In2 : Inport  Port=4  PortName=InBus1
  Bus Element In1 : Inport  Port=5  PortName=BstPetFile
  Bus Element In3 : Inport  Port=6  PortName=InBus2
  Bus Element In9 : Inport  Port=7  PortName=InBus8
  Bus Element Out1 : Outport  PortName=PetFile
  Bus Element Out3 : Outport  Port=2  PortName=OutBus1
  Bus Element Out2 : Outport  Port=3  PortName=OutBus
  Bus Element Out4 : Outport  Port=4  PortName=OutBus2
  Bus Element Out5 : Outport  Port=5  PortName=OutBus3
  Bus Element Out8 : Outport  Port=6  PortName=OutBus6
  Bus Element Out6 : Outport  Port=7  PortName=OutBus5

== system pet_logical_architecture/Data Storage/T1w MRI in Nifti or MGZ ==

== system pet_logical_architecture/GUI/Brainstorm GUI  ==
  PET Icon in Brainstorm Tree : Subsystem
      settings: PortSchema="{\"entries\":[{\"content\":{\"headerSize\":26,\"margin\":15,\"minimumSpacing\":25,\"sides\":[{\"content\":{},\"type\":\"ConnectorPlacement.EquallySpacedRectSide\",\"uuid\":\"41d3ebd7-d990-4c64-a8fe-a1444a13acba\"},{\"content\":{\"side\":\"RIGHT\"},\"type\":\"ConnectorPlacement.EquallySpacedRectSide\",\"uuid\":\"34a032e5-8bdc-4c16-a398-56e9e8002181\"},{\"content\":{\"side\":\"TOP\"},\"type\":\"ConnectorPlacement.EquallySpacedRectSide\",\"uuid\":\"d28171cf-e891-45d3-8ea9-b10c38c32c2e\"}]},\"type\":\"ConnectorPlacement.EquallySpacedConnector\",\"uuid\":\"0daa939b-8979-496f-bab9-c42cbb494216\"}],\"packageUris\":[\"http://schema.mathworks.com/mf0/Connector/R2020b\"],\"version\":\"1.0\"}"

== system pet_logical_architecture/GUI/MRI Viewer ==

== system pet_logical_architecture/GUI/PET Autoprocess ==

== system pet_logical_architecture/GUI/PET Processing Utility ==

== system pet_logical_architecture/I//O /Import PET ==

== system pet_logical_architecture/I//O /Load Existing Protocol ==

== system pet_logical_architecture/I//O /Save database ==

== system pet_logical_architecture/I//O /Save imported PET file ==

== system pet_logical_architecture/I//O /Update protocol with new PET ==

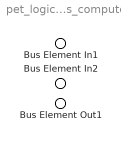
== system pet_logical_architecture/Pre-processor/cs_compute ==
  Bus Element In1 : Inport  PortName=PET
  Bus Element In2 : Inport  Port=2  PortName=vox2ras
  Bus Element Out1 : Outport  PortName=PetFile

== system pet_logical_architecture/Pre-processor/fs_align_pet ==
  Bus Element In1 : Inport  PortName=inVol
  Bus Element Out1 : Outport  PortName=fsPetFile

== system pet_logical_architecture/Pre-processor/fs_frame_mean ==
  Bus Element In1 : Inport  PortName=fsPetFile
  Bus Element Out1 : Outport  PortName=fsPet

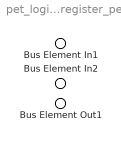
== system pet_logical_architecture/Pre-processor/fs_register_pet ==
  Bus Element In1 : Inport  PortName=fsPetFile
  Bus Element In2 : Inport  Port=2  PortName=mri_nii
  Bus Element Out1 : Outport  PortName=fsPet

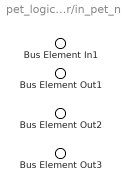
== system pet_logical_architecture/Pre-processor/in_pet_nii ==
  Bus Element In1 : Inport  PortName=PetFile
  Bus Element Out1 : Outport  PortName=PET
  Bus Element Out2 : Outport  Port=2  PortName=vox2ras
  Bus Element Out3 : Outport  Port=3  PortName=tReorient

== system pet_logical_architecture/Pre-processor/out_mri_nii ==
  Bus Element In1 : Inport  AllowServiceAccess=on  PortName=BstMriFile
  Bus Element Out1 : Outport  PortName=mri_nii

== system pet_logical_architecture/Pre-processor/tess_mri_mask ==
  Bus Element In1 : Inport  PortName=PetFile
  Bus Element Out1 : Outport  PortName=OutBus

== system pet_logical_architecture/Processor/PVC  ==

== system pet_logical_architecture/Processor/SUVR ==

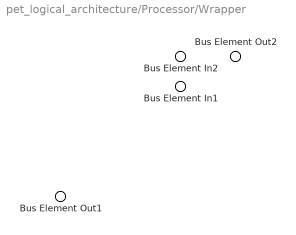
== system pet_logical_architecture/Processor/Wrapper ==
  Bus Element In1 : Inport  PortName=InBus
  Bus Element In2 : Inport  Port=2  PortName=InBus1
  Bus Element Out2 : Outport  PortName=OutBus1
  Bus Element Out1 : Outport  Port=2  PortName=OutBus

== system pet_logical_architecture/GUI/Brainstorm GUI /PET Icon in Brainstorm Tree ==
